simulink model "farol"  (R2022a)
settings: Solver=VariableStepAuto  StartTime=0.0  StopTime=10.0  RelTol=1e-3
settings Model: Creator=Usuario  LastModifiedBy=Usuario

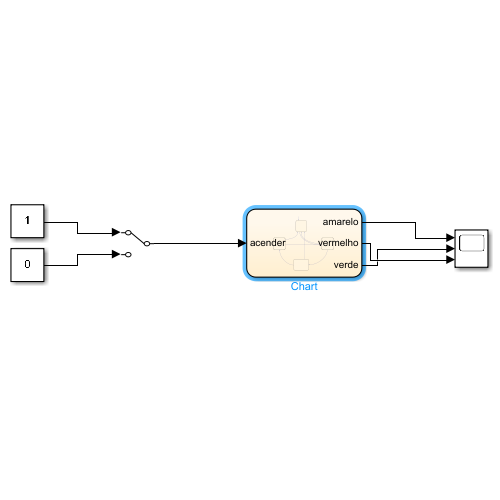
[thumbnail: Simulink's stored preview of the top-level diagram]
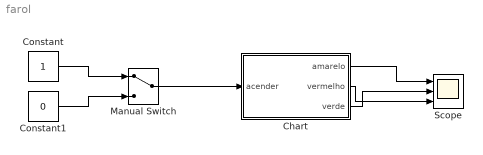
== system farol ==
  Chart : Stateflow chart  TreatAsAtomicUnit=on
  Constant : Constant  OutDataTypeStr=boolean
  Constant1 : Constant  Value=0  OutDataTypeStr=boolean
  Manual Switch : ManualSwitch
  Scope : Scope  NumInputPorts=3
  wires:
  Constant/1 -> Manual Switch/1
  Constant1/1 -> Manual Switch/2
  Manual Switch/1 -> Chart/1(acender)
  Chart/1(amarelo) -> Scope/1
  Chart/2(vermelho) -> Scope/3
  Chart/3(verde) -> Scope/2

== stateflow chart farol/Chart ==
  state acender
    entry:
    vermelho =0;
    amarelo = 0;
    verde =0;
  state amarelo
    entry:
    vermelho = 0;
    amarelo = 1;
    verde = 0;
  state vermelho
    entry:
    vermelho = 1;
    amarelo = 0;
    verde = 0;
  state verde
    entry:
    vermelho = 0;
    amarelo = 0;
    verde = 1;
  (default) -> acender
  amarelo -> acender [order 2] : [acender ==0]
  acender -> vermelho : [acender ==1]
  vermelho -> acender [order 2] : [acender ==0]
  verde -> acender [order 2] : [acender ==0]
  amarelo -> vermelho [order 1] : after(2,sec)
  verde -> amarelo [order 1] : after(2,sec)
  vermelho -> verde [order 1] : after(2,sec)
  data: amarelo output; vermelho output; verde output; acender input
